simulink model "DCmachine_sim"  (R2023b)
settings: Solver=VariableStepAuto  StartTime=0.0  StopTime=700  RelTol=1e-3
values from neighbouring files (symbols this model uses):
  an = 60*(1000/3600)/25    (= 0.666666666667)    [DCmachine.m]
  beta = Tf/wn    (= 0.976675486798)    [DCmachine.m]
  En = Pn/Ian    (= 540)    [DCmachine.m]
  Ien = 1    [DCmachine.m]
  J = M*R^2    (= 73.2506615098)    [DCmachine.m]
  Ks = Tn/(Ian*Ien)    (= 1.71974522293)    [DCmachine.m]
  La = tau_a*Ra    (= 0.00084)    [DCmachine.m]
  Le = tau_e*Re    (= 120)    [DCmachine.m]
  M = 10*1000+200*80    (= 26000)    [DCmachine.m]
  R = vn/wn    (= 0.0530785562633)    [DCmachine.m]
  Ra = 0.084    [DCmachine.m]
  Re = Ven/Ien    (= 120)    [DCmachine.m]
  Tn = Pn/wn    (= 1226.70441142)    [DCmachine.m]
  Van = 600    [DCmachine.m]
  Ven = 120    [DCmachine.m]
  wn = 314    [DCmachine.m]
undefined symbols (not defined in the file or in its folder): Reg_Iapi, Reg_Iepi, Reg_wpi
libraries: slpidlib x2, simulink x1
settings Model: Creator=lollo  LastModifiedBy=lollo

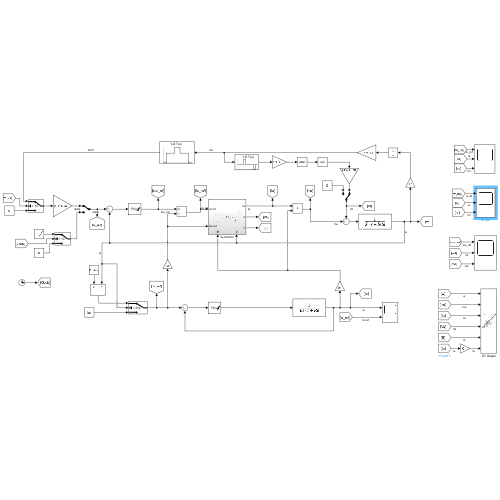
[thumbnail: Simulink's stored preview of the top-level diagram]
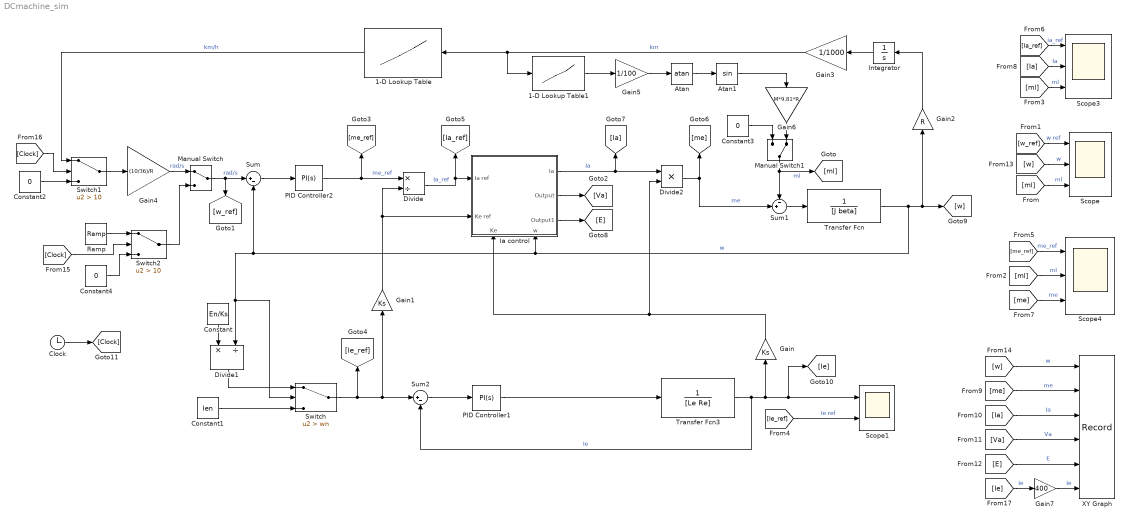
== system DCmachine_sim ==
  1-D Lookup Table : Lookup_n-D  NumberOfTableDimensions=1  BreakpointsForDimension1=[0;1;1.001;4;4.001;6;6.001;9;9.001;10]  Table=[35;35;60;60;75;75;60;60;35;35]  InternalRulePriority=Speed  RndMeth=Simplest
  1-D Lookup Table1 : Lookup_n-D  NumberOfTableDimensions=1  BreakpointsForDimension1=[0;3;3.001;4;4.001;8;8.001;9;9.001;10]  Table=[0;0;5;5;0;0;-5;-5;0;0]  InternalRulePriority=Speed  RndMeth=Simplest
  Atan : Trigonometry  Operator=atan
  Atan1 : Trigonometry
  Clock : Clock
  Constant : Constant  Value=En/Ks
  Constant1 : Constant  Value=Ien
  Constant2 : Constant  Value=0
  Constant3 : Constant  Value=0
  Constant4 : Constant  Value=0
  Divide : Product  Inputs=*/
  Divide1 : Product  Inputs=*/
  Divide2 : Product  Inputs=**
  Gain : Gain  Gain=Ks
  Gain1 : Gain  Gain=Ks
  Gain2 : Gain  Gain=R
  Gain3 : Gain  Gain=1/1000
  Gain4 : Gain  Gain=(10/36)/R
  Gain5 : Gain  Gain=1/100
  Gain6 : Gain  Gain=M*9.81*R
  Gain7 : Gain  Gain=400
  Ia control : Subsystem
      settings: PortSchema="{\"entries\":[{\"content\":{\"sides\":[{\"content\":{\"connectorIds\":[\"In1\",\"In2\"]},\"type\":\"ConnectorPlacement.EquallySpacedRectSide\",\"uuid\":\"ec57bc2f-c43b-4541-b3f5-963951984ff0\"},{\"content\":{\"connectorIds\":[\"Out1\",\"Out2\",\"Out3\"],\"side\":\"RIGHT\"},\"type\":\"ConnectorPlacement.EquallySpacedRectSide\",\"uuid\":\"d5bae3d5-17a3-4c12-bded-28f17bd9faef\"},{\"content\":{\"side\":\"TOP\"},\"type\":\"ConnectorPlacement.EquallySpacedRectSide\",\"uuid\":\"d2e0a3dc-5acf-48dc-9d94-768bccada07b\"},{\"content\":{\"connectorIds\":[\"In3\",\"In4\"],\"side\":\"BOTTOM\"},\"type\":\"ConnectorPlacement.EquallySpacedRectSide\",\"uuid\":\"e46819b1-4823-4918-bb2a-a4d51449290e\"}]},\"type\":\"ConnectorPlacement.EquallySpacedConnector\",\"uuid\":\"93bdb7b4-54f4-4037-9248-ecfd17b8235b\"}],\"packageUris\":[\"http://schema.mathworks.com/mf0/Connector/R2020b\"],\"version\":\"1.0\"}"
  Integrator : Integrator
  Manual Switch : ManualSwitch
  Manual Switch1 : ManualSwitch  CurrentSetting=0
  PID Controller1 : slpidlib/PID Controller  Controller=PI  Form=Parallel  TimeDomain=Continuous-time  UseExternalTs=off  SampleTime=-1  IntegratorMethod=Forward Euler  FilterMethod=Forward Euler  ControllerParametersSource=internal  P=Reg_Iepi.Kp  I=Reg_Iepi.Ki  UseKiTs=off  D=0  N=100  UseFilter=on  TunerSelectOption=Transfer Function Based (PID Tuner App)  InitialConditionSource=internal  InitialConditionForIntegrator=0  InitialConditionForFilter=0  DifferentiatorICPrevScaledInput=0  ExternalReset=none  TrackingMode=off  Kt=1  LimitOutput=on  SatLimitsSource=internal  UpperSaturationLimit=Ven  LowerSaturationLimit=-Ven  LinearizeAsGain=on  AntiWindupMode=back-calculation  Kb=Reg_Iepi.Ki  LimitIntegrator=off  UpperIntegratorSaturationLimit=inf  LowerIntegratorSaturationLimit=-inf  POutMin=[]  POutMax=[]  IOutMin=[]  IOutMax=[]  DOutMin=[]  DOutMax=[]  NOutMin=[]  NOutMax=[]  SumOutMin=[]  SumOutMax=[]  SaturationOutMin=[]  SaturationOutMax=[]  PParamMin=[]  PParamMax=[]  IParamMin=[]  IParamMax=[]  DParamMin=[]  DParamMax=[]  NParamMin=[]  NParamMax=[]  KbParamMin=[]  KbParamMax=[]  KtParamMin=[]  KtParamMax=[]  KbOutMin=[]  KbOutMax=[]  KtOutMin=[]  KtOutMax=[]  IntegratorOutMin=[]  IntegratorOutMax=[]  FilterOutMin=[]  FilterOutMax=[]  SumI1OutMin=[]  SumI1OutMax=[]  SumI2OutMin=[]  SumI2OutMax=[]  SumI3OutMin=[]  SumI3OutMax=[]  SumI4OutMin=[]  SumI4OutMax=[]  SumDOutMin=[]  SumDOutMax=[]  DifferentiatorOutMin=[]  DifferentiatorOutMax=[]  FilterDiffOutCoefMin=[]  FilterDiffOutCoefMax=[]  ReciprocalOutMin=[]  ReciprocalOutMax=[]  SumDenOutMin=[]  SumDenOutMax=[]  SumNumOutMin=[]  SumNumOutMax=[]  DivideOutMin=[]  DivideOutMax=[]  UdiffTsProdOutMin=[]  UdiffTsProdOutMax=[]  NTsProdOutMin=[]  NTsProdOutMax=[]  UintegralTsProdOutMin=[]  UintegralTsProdOutMax=[]  UngainTsProdOutMin=[]  UngainTsProdOutMax=[]  ClampingZeroOutDataTypeStr=Inherit: Inherit via back propagation  ClampingZeroOutMin=[]  ClampingZeroOutMax=[]  FilterDenConstantOutDataTypeStr=Inherit: Inherit via back propagation  FilterDenConstantOutMin=[]  FilterDenConstantOutMax=[]  PCopyOutDataTypeStr=Inherit: Inherit via back propagation  PCopyOutMin=[]  PCopyOutMax=[]  NCopyOutDataTypeStr=Inherit: Inherit via back propagation  NCopyOutMin=[]  NCopyOutMax=[]  IntegratorContinuousStateAttributes=''  IntegratorStateMustResolveToSignalObject=off  IntegratorRTWStateStorageClass=Auto  FilterContinuousStateAttributes=''  FilterStateMustResolveToSignalObject=off  FilterRTWStateStorageClass=Auto  ParallelPVariant=InternalParameters  IdealPVariant=Disabled  IVariant=InternalParameters  DVariant=Disabled  IntegratorVariant=Continuous  SatVariant=Enabled  AWVariant=BackCalculation  PCopyVariant=Disabled  TRVariant=Disabled  FdbkBlocksVariant=Forward  IdealPFdbkVariant=Disabled  SatFdbkVariant=Disabled  DerivativeFilterVariant=Disabled  NVariant=Disabled  NCopyVariant=Disabled_SignalSpec  FilterICVariant=Disabled  IntegratorICVariant=InternalICs  ExternalResetVariant=Disabled  TRSumVariant=Passthrough  SumFdbkVariant=Disabled  SumVariant=Sum_PI  TsampFilterVariant=InternalTs  TsampNgainVariant=Passthrough  TsampIntegralVariant=Disabled_SignalSpec  ExternalSaturationOutDataTypeStr=Inherit: Same as second input
  PID Controller2 : slpidlib/PID Controller  Controller=PI  Form=Parallel  TimeDomain=Continuous-time  UseExternalTs=off  SampleTime=-1  IntegratorMethod=Forward Euler  FilterMethod=Forward Euler  ControllerParametersSource=internal  P=Reg_wpi.Kp  I=Reg_wpi.Ki  UseKiTs=off  D=Reg_wpi.Kd  N=100  UseFilter=on  TunerSelectOption=Transfer Function Based (PID Tuner App)  InitialConditionSource=internal  InitialConditionForIntegrator=0  InitialConditionForFilter=0  DifferentiatorICPrevScaledInput=0  ExternalReset=none  TrackingMode=off  Kt=1  LimitOutput=on  SatLimitsSource=internal  UpperSaturationLimit=1400  LowerSaturationLimit=-1400  LinearizeAsGain=on  AntiWindupMode=back-calculation  Kb=0.08  LimitIntegrator=off  UpperIntegratorSaturationLimit=Tn  LowerIntegratorSaturationLimit=-Tn  POutMin=[]  POutMax=[]  IOutMin=[]  IOutMax=[]  DOutMin=[]  DOutMax=[]  NOutMin=[]  NOutMax=[]  SumOutMin=[]  SumOutMax=[]  SaturationOutMin=[]  SaturationOutMax=[]  PParamMin=[]  PParamMax=[]  IParamMin=[]  IParamMax=[]  DParamMin=[]  DParamMax=[]  NParamMin=[]  NParamMax=[]  KbParamMin=[]  KbParamMax=[]  KtParamMin=[]  KtParamMax=[]  KbOutMin=[]  KbOutMax=[]  KtOutMin=[]  KtOutMax=[]  IntegratorOutMin=[]  IntegratorOutMax=[]  FilterOutMin=[]  FilterOutMax=[]  SumI1OutMin=[]  SumI1OutMax=[]  SumI2OutMin=[]  SumI2OutMax=[]  SumI3OutMin=[]  SumI3OutMax=[]  SumI4OutMin=[]  SumI4OutMax=[]  SumDOutMin=[]  SumDOutMax=[]  DifferentiatorOutMin=[]  DifferentiatorOutMax=[]  FilterDiffOutCoefMin=[]  FilterDiffOutCoefMax=[]  ReciprocalOutMin=[]  ReciprocalOutMax=[]  SumDenOutMin=[]  SumDenOutMax=[]  SumNumOutMin=[]  SumNumOutMax=[]  DivideOutMin=[]  DivideOutMax=[]  UdiffTsProdOutMin=[]  UdiffTsProdOutMax=[]  NTsProdOutMin=[]  NTsProdOutMax=[]  UintegralTsProdOutMin=[]  UintegralTsProdOutMax=[]  UngainTsProdOutMin=[]  UngainTsProdOutMax=[]  ClampingZeroOutDataTypeStr=Inherit: Inherit via back propagation  ClampingZeroOutMin=[]  ClampingZeroOutMax=[]  FilterDenConstantOutDataTypeStr=Inherit: Inherit via back propagation  FilterDenConstantOutMin=[]  FilterDenConstantOutMax=[]  PCopyOutDataTypeStr=Inherit: Inherit via back propagation  PCopyOutMin=[]  PCopyOutMax=[]  NCopyOutDataTypeStr=Inherit: Inherit via back propagation  NCopyOutMin=[]  NCopyOutMax=[]  IntegratorContinuousStateAttributes=''  IntegratorStateMustResolveToSignalObject=off  IntegratorRTWStateStorageClass=Auto  FilterContinuousStateAttributes=''  FilterStateMustResolveToSignalObject=off  FilterRTWStateStorageClass=Auto  ParallelPVariant=InternalParameters  IdealPVariant=Disabled  IVariant=InternalParameters  DVariant=Disabled  IntegratorVariant=Continuous  SatVariant=Enabled  AWVariant=BackCalculation  PCopyVariant=Disabled  TRVariant=Disabled  FdbkBlocksVariant=Forward  IdealPFdbkVariant=Disabled  SatFdbkVariant=Disabled  DerivativeFilterVariant=Disabled  NVariant=Disabled  NCopyVariant=Disabled_SignalSpec  FilterICVariant=Disabled  IntegratorICVariant=InternalICs  ExternalResetVariant=Disabled  TRSumVariant=Passthrough  SumFdbkVariant=Disabled  SumVariant=Sum_PI  TsampFilterVariant=InternalTs  TsampNgainVariant=Passthrough  TsampIntegralVariant=Disabled_SignalSpec  ExternalSaturationOutDataTypeStr=Inherit: Same as second input
  Ramp : simulink/Sources/Ramp  slope=an/R  start=10  InitialOutput=0
  Scope : Scope  NumInputPorts=3
  Scope1 : Scope  NumInputPorts=2
  Scope3 : Scope  NumInputPorts=3
  Scope4 : Scope  NumInputPorts=3
  Sum : Sum  Inputs=|+-
  Sum1 : Sum  Inputs=-+|
  Sum2 : Sum  Inputs=|+-
  Switch : Switch  Criteria=u2 > Threshold  Threshold=wn  SaturateOnIntegerOverflow=off  InputSameDT=off
  Switch1 : Switch  Criteria=u2 > Threshold  Threshold=10  SaturateOnIntegerOverflow=off  InputSameDT=off
  Switch2 : Switch  Criteria=u2 > Threshold  Threshold=10  SaturateOnIntegerOverflow=off  InputSameDT=off
  Transfer Fcn : TransferFcn  Denominator=[J beta]
  Transfer Fcn3 : TransferFcn  Denominator=[Le Re]
  XY Graph : Record  FileSettingsInternal="{\"entries\":[{\"content\":{\"excelSettings\":{\"content\":{},\"type\":\"Streamout.ExcelSettings\"}},\"type\":\"Streamout.FileSettingStorage\",\"uuid\":\"\"}],\"packageUris\":[\"http:\\/\\/schema.mathworks.com\\/mf0\\/streamout_blocks\\/R2020a\"],\"version\":\"1.0\"}"  Layout=[1 1]  SignalsInternal="{\"entries\":[{\"content\":{\"signals\":[{\"content\":{\"blockPath\":[],\"dimensions\":[1],\"domain\":\"\",\"lineColor\":\"#a2142f\",\"plots\":[ 1, 9 ],\"port\":1,\"sid\":[\"\"],\"signalID\":1,\"signalName\":\"w\"},\"type\":\"RecordBlkView.Signal\",\"uuid\":\"\"},{\"content\":{\"blockPath\":[],\"dimensions\":[1],\"domain\":\"\",\"lineColor\":\"#edb120\",\"plots\":[ 1, 9 ],\"port\":2,\"sid\":[\"\"],\"signalID\":2,\"signalName\":\"me\"},\"type\":\"RecordBlkView.Signal\",\"uuid\":\"\"},{\"content\":{\"blockPath\":[],\"dimensions\":[1],\"domain\":\"\",\"lineColor\":\"#ff6929\",\"plots\":[ 1, 9 ],\"port\":3,\"sid\":[\"\"],\"signalID\":3,\"signalName\":\"Ia\"},\"type\":\"RecordBlkView.Signal\",\"uuid\":\"\"},{\"content\":{\"blockPath\":[],\"dimensions\":[1],\"domain\":\"\",\"lineColor\":\"#a2142f\",\"plots\":[ 1, 9 ],\"port\":4,\"sid\":[\"\"],\"signalID\":4,\"signalName\":\"Va\"},\"type\":\"RecordBlkView.Signal\",\"uuid\":\"\"},{\"content\":{\"blockPath\":[],\"dimensions\":[1],\"domain\":\"\",\"lineColor\":\"#139fff\",\"plots\":[ 1, 9 ],\"port\":5,\"sid\":[\"\"],\"signalID\":5,\"signalName\":\"E\"},\"type\":\"RecordBlkView.Signal\",\"uuid\":\"\"},{\"content\":{\"blockPath\":[],\"dimensions\":[1],\"domain\":\"\",\"lineColor\":\"#d95319\",\"plots\":[ 1 ],\"port\":6,\"sid\":[\"\"],\"signalID\":6,\"signalName\":\"Ie\"},\"type\":\"RecordBlkView.Signal\",\"uuid\":\"\"}]},\"type\":\"RecordBlkView.InputSignals\",\"uuid\":\"\"}],\"packageUris\":[\"http:\\/\\/schema.mathworks.com\\/mf0\\/streamout_blocks\\/R2020a\"],\"version\":\"1.0\"}"  VisualizationBindings="{\"xyplotplugin\":{\"info\":[{\"series\":[{\"bindingParametersList\":[{\"parameter\":\"X-Axis\",\"signalID\":1,\"signalName\":\"w\"},{\"parameter\":\"Y-Axis\",\"signalID\":3,\"signalName\":\"Ia\"},{\"parameter\":\"X-Axis\",\"signalID\":1,\"signalName\":\"w\"},{\"parameter\":\"Y-Axis\",\"signalID\":3,\"signalName\":\"Ia\"}],\"seriesID\":0},{\"bindingParametersList\":[{\"parameter\":\"X-Axis\",\"signalID\":1,\"signalName\":\"w\"},{\"parameter\":\"Y-Axis\",\"signalID\":5,\"signalName\":\"E\"},{\"parameter\":\"X-Axis\",\"signalID\":1,\"signalName\":\"w\"},{\"parameter\":\"Y-Axis\",\"signalID\":5,\"signalName\":\"E\"}],\"seriesID\":1},{\"bindingParametersList\":[{\"parameter\":\"X-Axis\",\"signalID\":1,\"signalName\":\"w\"},{\"parameter\":\"Y-Axis\",\"signalID\":4,\"signalName\":\"Va\"},{\"parameter\":\"X-Axis\",\"signalID\":1,\"signalName\":\"w\"},{\"parameter\":\"Y-Axis\",\"signalID\":4,\"signalName\":\"Va\"}],\"seriesID\":2},{\"bindingParametersList\":[{\"parameter\":\"X-Axis\",\"signalID\":1,\"signalName\":\"w\"},{\"parameter\":\"Y-Axis\",\"signalID\":2,\"signalName\":\"me\"},{\"parameter\":\"X-Axis\",\"signalID\":1,\"signalName\":\"w\"},{\"parameter\":\"Y-Axis\",\"signalID\":2,\"signalName\":\"me\"}],\"seriesID\":3},{\"bindingParametersList\":[{\"parameter\":\"X-Axis\",\"signalID\":1,\"signalName\":\"w\"},{\"parameter\":\"Y-Axis\",\"signalID\":6,\"signalName\":\"Ie\"}],\"seriesID\":4}],\"subplotID\":1},{\"series\":[{\"bindingParametersList\":[{\"parameter\":\"X-Axis\",\"signalID\":1,\"signalName\":\"w\"},{\"parameter\":\"Y-Axis\",\"signalID\":2,\"signalName\":\"me\"}],\"seriesID\":5},{\"bindingParametersList\":[{\"parameter\":\"X-Axis\",\"signalID\":1,\"signalName\":\"w\"},{\"parameter\":\"Y-Axis\",\"signalID\":4,\"signalName\":\"Va\"}],\"seriesID\":6},{\"bindingParametersList\":[{\"parameter\":\"X-Axis\",\"signalID\":1,\"signalName\":\"w\"},{\"parameter\":\"Y-Axis\",\"signalID\":3,\"signalName\":\"Ia\"}],\"seriesID\":7},{\"bindingParametersList\":[{\"parameter\":\"X-Axis\",\"signalID\":1,\"signalName\":\"w\"},{\"parameter\":\"Y-Axis\",\"signalID\":5,\"signalName\":\"E\"}],\"seriesID\":8}],\"subplotID\":9}]}}"  CompatibilityTag=XY
  wires:
  Sum/1 -> PID Controller2/1
  PID Controller2/1 -> Divide/1, [me_ref]  "me_ref"
  Constant/1 -> Divide1/1
  Switch/1 -> Sum2/1, Gain1/1, [Ie_ref]
  Gain1/1 -> Divide/2, Ia control/2(Ke ref)
  Sum2/1 -> PID Controller1/1
  PID Controller1/1 -> Transfer Fcn3/1
  Transfer Fcn3/1 -> Gain/1, [Ie], Scope1/1, Sum2/2  "Ie"
  Transfer Fcn/1 -> Switch/2, Divide1/2, Sum/2, Ia control/4(w), [w], Gain2/1  "w"
  Gain/1 -> Ia control/3(Ke), Divide2/2
  Sum1/1 -> Transfer Fcn/1
  1-D Lookup Table1/1 -> Gain5/1
  [w_ref] -> Scope/1  "w ref"
  [Ie_ref] -> Scope1/2  "Ie ref"
  Constant1/1 -> Switch/3
  Divide1/1 -> Switch/1
  Divide2/1 -> Sum1/2, [me]  "me"
  Gain2/1 -> Integrator/1
  Integrator/1 -> Gain3/1
  Gain3/1 -> 1-D Lookup Table/1, 1-D Lookup Table1/1  "km"
  Switch1/1 -> Gain4/1
  Constant2/1 -> Switch1/3
  1-D Lookup Table/1 -> Switch1/1  "km/h"
  Manual Switch/1 -> Sum/1, [w_ref]  "rad/s"
  Gain5/1 -> Atan/1
  Atan/1 -> Atan1/1
  Atan1/1 -> Gain6/1
  Gain6/1 -> Manual Switch1/2
  [ml] -> Scope/3  "ml"
  Divide/1 -> [Ia_ref], Ia control/1(Ia ref)  "Ia_ref"
  Ia control/1(Ia) -> Divide2/1, [Ia]  "Ia"
  [Ia] -> Scope3/2  "Ia"
  [ml] -> Scope3/3  "ml"
  [Ia_ref] -> Scope3/1  "ia_ref"
  [me] -> Scope4/3  "me"
  [ml] -> Scope4/2  "ml"
  [me_ref] -> Scope4/1  "me_ref"
  Ramp/1 -> Switch2/1
  Gain4/1 -> Manual Switch/1  "rad/s"
  Ia control/2(Output) -> [Va]
  Manual Switch1/1 -> Sum1/1, [ml]  "ml"
  Constant3/1 -> Manual Switch1/1
  Switch2/1 -> Manual Switch/2
  Constant4/1 -> Switch2/3
  Ia control/3(Output1) -> [E]
  [E] -> XY Graph/5  "E"
  [me] -> XY Graph/2  "me"
  [Va] -> XY Graph/4  "Va"
  [Ia] -> XY Graph/3  "Ia"
  [w] -> XY Graph/1  "w"
  Clock/1 -> [Clock]
  [Clock] -> Switch1/2
  [Clock] -> Switch2/2
  [w] -> Scope/2  "w"
  [Ie] -> Gain7/1  "Ie"
  Gain7/1 -> XY Graph/6  "Ie"

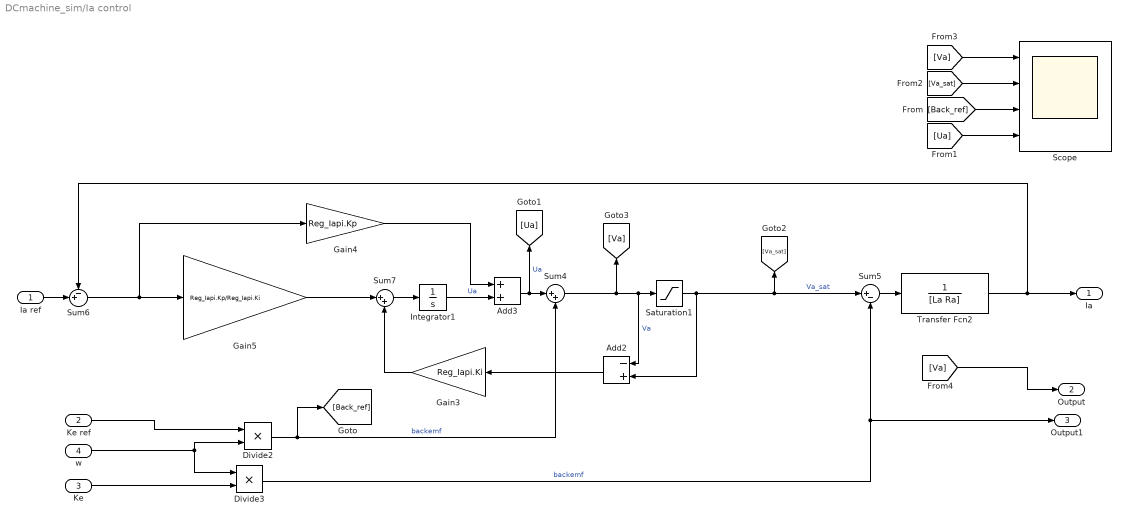
== system DCmachine_sim/Ia control ==
  Ia ref : Inport
  Ke ref : Inport  Port=2
  Ke : Inport  Port=3
  w : Inport  Port=4
  Add2 : Sum  Inputs=-+
  Add3 : Sum
  Divide2 : Product  Inputs=**
  Divide3 : Product  Inputs=**
  Gain3 : Gain  Gain=Reg_Iapi.Ki
  Gain4 : Gain  Gain=Reg_Iapi.Kp
  Gain5 : Gain  Gain=Reg_Iapi.Kp/Reg_Iapi.Ki
  Integrator1 : Integrator
  Saturation1 : Saturate  UpperLimit=Van  LowerLimit=-Van
  Scope : Scope  NumInputPorts=4
  Sum4 : Sum  Inputs=|++
  Sum5 : Sum  Inputs=|+-
  Sum6 : Sum  Inputs=-+|
  Sum7 : Sum  Inputs=|++
  Transfer Fcn2 : TransferFcn  Denominator=[La Ra]
  Ia : Outport
  Output : Outport  Port=2
  Output1 : Outport  Port=3
  wires:
  Add2/1 -> Gain3/1
  Integrator1/1 -> Add3/2  "Ua"
  Gain3/1 -> Sum7/2
  Gain5/1 -> Sum7/1
  Sum6/1 -> Gain4/1, Gain5/1
  Sum7/1 -> Integrator1/1
  Gain4/1 -> Add3/1
  Divide3/1 -> Sum5/2, Output1/1  "backemf"
  Divide2/1 -> [Back_ref], Sum4/2  "backemf"
  Add3/1 -> Sum4/1, [Ua]  "Ua"
  Sum5/1 -> Transfer Fcn2/1
  Sum4/1 -> Add2/1, Saturation1/1, [Va]  "Va"
  Transfer Fcn2/1 -> Ia/1, Sum6/1
  Ia ref/1 -> Sum6/2
  Ke ref/1 -> Divide2/1
  w/1 -> Divide2/2, Divide3/1
  Ke/1 -> Divide3/2
  Saturation1/1 -> Add2/2, [Va_sat], Sum5/1  "Va_sat"
  [Back_ref] -> Scope/3
  [Ua] -> Scope/4
  [Va_sat] -> Scope/2
  [Va] -> Scope/1
  [Va] -> Output/1
